simulink model "Closedloop"  (R2015b)
settings: Solver=VariableStepAuto  StartTime=0.0  StopTime=100  FixedStep=0.0001  RelTol=1e-6
values from neighbouring files (symbols this model uses):
  A = [a11 a12 a13;a21 a22 a23;a31 a32 a33]    [ControllerWT1.m]    (also in ControllerWT2.m; Robustness.m)
  B = [b11*10^6 b12*10^4;b21*10^6 b22*10^4;b31*10^6 b32*10^4]    [ControllerWT1.m]    (also in ControllerWT2.m; Robustness.m = [0 b11*10^6 b12*10^4;0 b21*10^6 b22*10^4;0 b31*10^6 b32*10^4)
  C = [0 0 0;1 0 0;a21 a22 a23;0 0 0;0 1 0]    [ControllerWT1.m]    (also in ControllerWT2.m; Robustness.m = [0 0 0;1 0 0;a21 a22 a23;1 0 0;0 0 0;0 1 0])
  Cp = xlsread(filename)    [Run_me.m]
  D = [0 1;0 0;b21*10^6 b22*10^4;1 0;0 0]    [ControllerWT1.m]    (also in ControllerWT2.m; Robustness.m = [0 0 1;0 0 0;0 b21*10^6 b22*10^4;-lambda_opt/R 0 0;0 1 0;0 0)
  lambda_opt = 7.1    [ControllerWT1.m]    (also in ControllerWT2.m; Robustness.m; Run_me.m)
  R = ureal('Rho',35,'Percentage',1)    [ControllerWT1.m]    (also in ControllerWT2.m; Robustness.m = ureal('Rho',35,'Percentage',15); Run_me.m = 35)
  Rho = ureal('Rho',1.225,'Percentage',1)    [ControllerWT1.m]    (also in ControllerWT2.m; Robustness.m = ureal('Rho',1.225,'Percentage',15); Run_me.m = 1.225)
undefined symbols (not defined in the file or in its folder): OutList, strmatch
settings Model: Creator=bjonkman  LastModifiedBy=alino
settings DataIOCC: SaveFormat=Array  SignalLoggingSaveFormat=ModelDataLogs  SaveOutput=off  SaveTime=off  SignalLoggingName=sigsOut
settings OptimizationCC: ExpressionDepthLimit=2147483647
settings DebuggingCC: SaveWithParameterizedLinksMsg=none  UnderspecifiedInitializationDetection=Classic  MergeDetectMultiDrivingBlocksExec=none  SignalResolutionControl=TryResolveAllWithWarning  MultiTaskDSMMsg=warning  MultiTaskCondExecSysMsg=none  FcnCallInpInsideContextMsg=EnableAllAsWarning  StateNameClashWarn=warning
settings HardwareCC: ProdBitPerPointer=32  ProdLargestAtomicFloat=None  ProdIntDivRoundTo=Undefined  ProdEndianess=Unspecified  ProdWordSize=32  ProdHWDeviceType=32-bit Generic  TargetUnknown=on
settings GRTTargetCC: GeneratePreprocessorConditionals=Disable all  CombineOutputUpdateFcns=off  GRTInterface=on
settings ConfigComp: CovModelRefEnable=Off

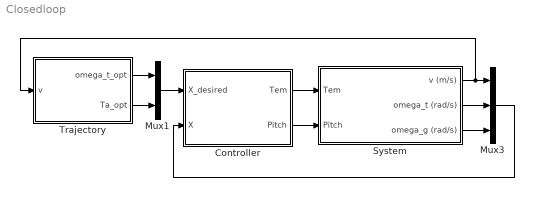
== system Closedloop ==
  Controller : Subsystem
  Mux1 : Mux  Inputs=2
  Mux3 : Mux  Inputs=3
  System : Subsystem
  Trajectory : Subsystem
  wires:
  Mux3/1 -> Controller/2(X)
  Mux1/1 -> Controller/1(X_desired)
  Trajectory/1(omega_t_opt) -> Mux1/1
  Controller/1(Tem) -> System/1(Tem)
  Controller/2(Pitch) -> System/2(Pitch)
  System/3(omega_g (rad/s)) -> Mux3/3
  System/2(omega_t (rad/s)) -> Mux3/2
  System/1(v (m/s)) -> Mux3/1, Trajectory/1(v)
  Trajectory/2(Ta_opt) -> Mux1/2

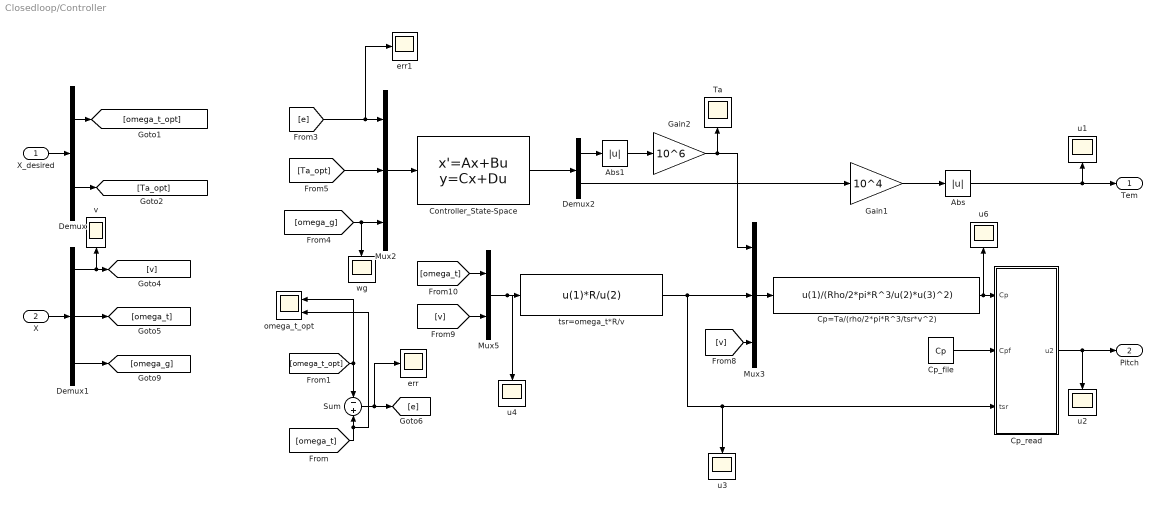
== system Closedloop/Controller ==
  X_desired : Inport
  X : Inport  Port=2
  Abs : Abs
  Abs1 : Abs
  Controller_State-Space : StateSpace  A=A  B=B  C=C  D=D  X0=0
  Cp=Ta/(rho/2*pi*R^3/tsr*v^2) : Fcn  Expr=u(1)/(Rho/2*pi*R^3/u(2)*u(3)^2)
  Cp_file : Constant  Value=Cp
  Cp_read : MATLAB Function  TreatAsAtomicUnit=on
  Demux : Demux  Outputs=2
  Demux1 : Demux  Outputs=3
  Demux2 : Demux  Outputs=2
  Gain1 : Gain  Gain=10^4
  Gain2 : Gain  Gain=10^6
  Mux2 : Mux  Inputs=3
  Mux3 : Mux  Inputs=3
  Mux5 : Mux  Inputs=2
  Sum : Sum  Inputs=-+
  Ta : Scope
  err : Scope
  err1 : Scope
  omega_t_opt : Scope  NumInputPorts=2
  tsr=omega_t*R/v : Fcn  Expr=u(1)*R/u(2)
  u{1..4,6} (5 alike) : Scope
  v : Scope
  wg : Scope
  Tem : Outport
  Pitch : Outport  Port=2
  wires:
  X_desired/1 -> Demux/1
  X/1 -> Demux1/1
  Demux/1 -> [omega_t_opt]
  Demux/2 -> [Ta_opt]
  Demux1/1 -> v/1, [v]
  Demux1/2 -> [omega_t]
  Demux1/3 -> [omega_g]
  Cp_read/1(u2) -> u2/1, Pitch/1
  Sum/1 -> err/1, [e]
  [omega_t] -> omega_t_opt/2, Sum/2
  [omega_t_opt] -> omega_t_opt/1, Sum/1
  [v] -> Mux3/3
  Mux5/1 -> u4/1, tsr=omega_t*R/v/1
  [v] -> Mux5/2
  [omega_t] -> Mux5/1
  tsr=omega_t*R/v/1 -> Cp_read/3(tsr), u3/1, Mux3/2
  [omega_g] -> wg/1, Mux2/3
  [Ta_opt] -> Mux2/2
  Controller_State-Space/1 -> Demux2/1
  Gain2/1 -> Ta/1, Mux3/1
  Mux3/1 -> Cp=Ta/(rho/2*pi*R^3/tsr*v^2)/1
  Cp=Ta/(rho/2*pi*R^3/tsr*v^2)/1 -> u6/1, Cp_read/1(Cp)
  Cp_file/1 -> Cp_read/2(Cpf)
  Abs/1 -> u1/1, Tem/1
  [e] -> err1/1, Mux2/1
  Demux2/1 -> Abs1/1
  Demux2/2 -> Gain1/1
  Mux2/1 -> Controller_State-Space/1
  Gain1/1 -> Abs/1
  Abs1/1 -> Gain2/1

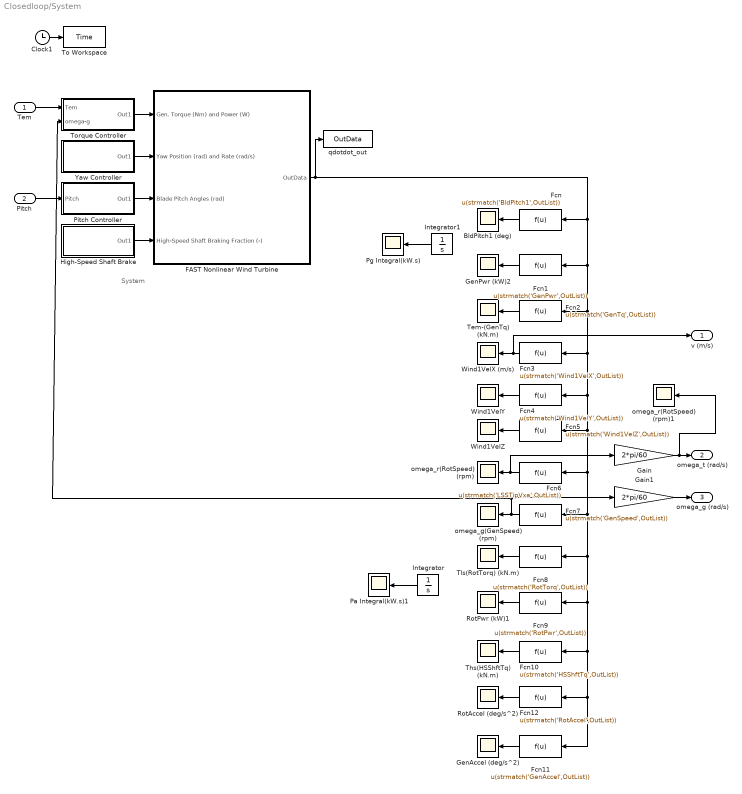
== system Closedloop/System ==
  note: System
  Tem : Inport
  Pitch : Inport  Port=2
  BldPitch1 (deg) : Scope
  Clock1 : Clock
  FAST Nonlinear Wind Turbine : Subsystem  mask(FAST Nonlinear Wind Turbine){}
      mask help: This block contains the FAST S-Function.
      mask init:
      | clear FAST_SFunc
  Fcn : Fcn  Expr=u(strmatch('BldPitch1',OutList))
  Fcn1 : Fcn  Expr=u(strmatch('GenPwr',OutList))
  Fcn10 : Fcn  Expr=u(strmatch('HSShftTq',OutList))
  Fcn11 : Fcn  Expr=u(strmatch('GenAccel',OutList))
  Fcn12 : Fcn  Expr=u(strmatch('RotAccel',OutList))
  Fcn2 : Fcn  Expr=u(strmatch('GenTq',OutList))
  Fcn3 : Fcn  Expr=u(strmatch('Wind1VelX',OutList))
  Fcn4 : Fcn  Expr=u(strmatch('Wind1VelY',OutList))
  Fcn5 : Fcn  Expr=u(strmatch('Wind1VelZ',OutList))
  Fcn6 : Fcn  Expr=u(strmatch('LSSTipVxa',OutList))
  Fcn7 : Fcn  Expr=u(strmatch('GenSpeed',OutList))
  Fcn8 : Fcn  Expr=u(strmatch('RotTorq',OutList))
  Fcn9 : Fcn  Expr=u(strmatch('RotPwr',OutList))
  Gain : Gain  Gain=2*pi/60
  Gain1 : Gain  Gain=2*pi/60
  GenAccel (deg/s^2) : Scope
  GenPwr (kW)2 : Scope
  High-Speed Shaft Brake : Subsystem
  Integrator : Integrator
  Integrator1 : Integrator
  Pa Integral(kW.s)1 : Scope
  Pg Integral(kW.s) : Scope
  Pitch Controller : Subsystem
  RotAccel (deg/s^2) : Scope
  RotPwr (kW)1 : Scope
  Tem-(GenTq) (kN.m) : Scope
  Ths(HSShftTq) (kN.m) : Scope
  Tls(RotTorq) (kN.m) : Scope
  To Workspace : ToWorkspace  VariableName=Time  SampleTime=-1
  Torque Controller : Subsystem
  Wind1VelX (m/s) : Scope
  Wind1VelY : Scope
  Wind1VelZ : Scope
  Yaw Controller : Subsystem
  omega_g(GenSpeed) (rpm) : Scope
  omega_r(RotSpeed) (rpm) : Scope
  omega_r(RotSpeed) (rpm)1 : Scope
  qdotdot_out : ToWorkspace  VariableName=OutData  SampleTime=-1
  v (m/s) : Outport
  omega_t (rad/s) : Outport  Port=2
  omega_g (rad/s) : Outport  Port=3
  wires:
  Clock1/1 -> To Workspace/1
  Torque Controller/1(Out1) -> FAST Nonlinear Wind Turbine/1(Gen. Torque (Nm) and Power (W))
  Yaw Controller/1(Out1) -> FAST Nonlinear Wind Turbine/2(Yaw Position (rad) and Rate (rad/s))
  Pitch Controller/1(Out1) -> FAST Nonlinear Wind Turbine/3(Blade Pitch Angles (rad))
  High-Speed Shaft Brake/1(Out1) -> FAST Nonlinear Wind Turbine/4(High-Speed Shaft Braking Fraction (-))
  Fcn/1 -> BldPitch1 (deg)/1
  Fcn2/1 -> Tem-(GenTq) (kN.m)/1
  Fcn3/1 -> v (m/s)/1, Wind1VelX (m/s)/1
  Fcn4/1 -> Wind1VelY/1
  Fcn5/1 -> Wind1VelZ/1
  Fcn6/1 -> Gain/1, omega_r(RotSpeed) (rpm)/1
  Fcn7/1 -> Torque Controller/2(omega-g), Gain1/1, omega_g(GenSpeed) (rpm)/1
  Fcn8/1 -> Tls(RotTorq) (kN.m)/1
  Fcn9/1 -> RotPwr (kW)1/1
  Fcn10/1 -> Ths(HSShftTq) (kN.m)/1
  Fcn12/1 -> RotAccel (deg/s^2)/1
  FAST Nonlinear Wind Turbine/1(OutData) -> Fcn11/1, Fcn12/1, Fcn10/1, Fcn9/1, Fcn8/1, Fcn7/1, Fcn6/1, Fcn5/1, Fcn4/1, Fcn3/1, Fcn2/1, Fcn1/1, Fcn/1, qdotdot_out/1
  Fcn11/1 -> GenAccel (deg/s^2)/1
  Tem/1 -> Torque Controller/1(Tem)
  Gain/1 -> omega_r(RotSpeed) (rpm)1/1, omega_t (rad/s)/1
  Gain1/1 -> omega_g (rad/s)/1
  Pitch/1 -> Pitch Controller/1(Pitch)
  Integrator/1 -> Pa Integral(kW.s)1/1
  Fcn1/1 -> GenPwr (kW)2/1
  Integrator1/1 -> Pg Integral(kW.s)/1

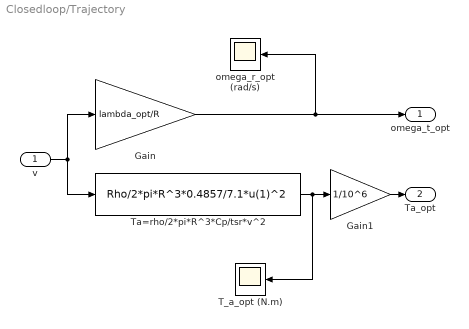
== system Closedloop/Trajectory ==
  v : Inport
  Gain : Gain  Gain=lambda_opt/R
  Gain1 : Gain  Gain=1/10^6
  T_a_opt (N.m) : Scope
  Ta=rho/2*pi*R^3*Cp/tsr*v^2 : Fcn  Expr=Rho/2*pi*R^3*0.4857/7.1*u(1)^2
  omega_r_opt (rad/s) : Scope
  omega_t_opt : Outport
  Ta_opt : Outport  Port=2
  wires:
  v/1 -> Gain/1, Ta=rho/2*pi*R^3*Cp/tsr*v^2/1
  Gain/1 -> omega_r_opt (rad/s)/1, omega_t_opt/1
  Gain1/1 -> Ta_opt/1
  Ta=rho/2*pi*R^3*Cp/tsr*v^2/1 -> T_a_opt (N.m)/1, Gain1/1

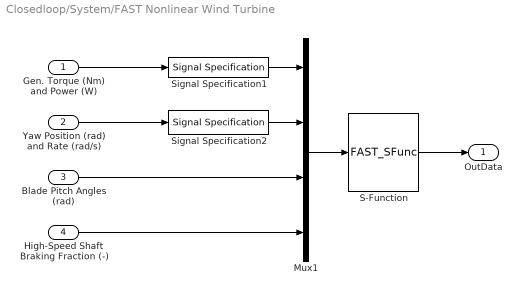
== system Closedloop/System/FAST Nonlinear Wind Turbine ==
  Gen. Torque (Nm) and Power (W) : Inport
  Yaw Position (rad) and Rate (rad/s) : Inport  Port=2
  Blade Pitch Angles (rad) : Inport  Port=3
  High-Speed Shaft Braking Fraction (-) : Inport  Port=4
  Mux1 : Mux
  S-Function : S-Function  FunctionName=FAST_SFunc  Parameters=FAST_InputFileName, TMax, 0  SFunctionDeploymentMode=off  EnableBusSupport=off
  Signal Specification1 : SignalSpecification  OutDataTypeStr=double  Dimensions=2
  Signal Specification2 : SignalSpecification  OutDataTypeStr=double  Dimensions=2
  OutData : Outport
  wires:
  Gen. Torque (Nm) and Power (W)/1 -> Signal Specification1/1
  S-Function/1 -> OutData/1
  Mux1/1 -> S-Function/1
  Blade Pitch Angles (rad)/1 -> Mux1/3
  Yaw Position (rad) and Rate (rad/s)/1 -> Signal Specification2/1
  Signal Specification1/1 -> Mux1/1
  Signal Specification2/1 -> Mux1/2
  High-Speed Shaft Braking Fraction (-)/1 -> Mux1/4

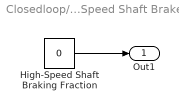
== system Closedloop/System/High-Speed Shaft Brake ==
  High-Speed Shaft Braking Fraction : Constant  Value=0
  Out1 : Outport
  wires:
  High-Speed Shaft Braking Fraction/1 -> Out1/1

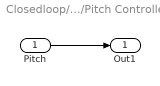
== system Closedloop/System/Pitch Controller ==
  Pitch : Inport
  Out1 : Outport
  wires:
  Pitch/1 -> Out1/1

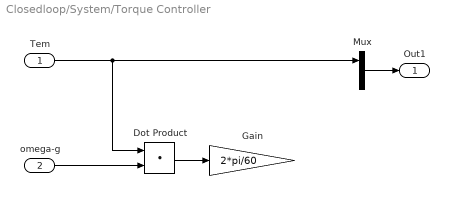
== system Closedloop/System/Torque Controller ==
  Tem : Inport
  omega-g : Inport  Port=2
  Dot Product : DotProduct  InputSameDT=on  OutDataTypeStr=Inherit: Inherit via internal rule
  Gain : Gain  Gain=2*pi/60
  Mux : Mux  Inputs=2
  Out1 : Outport
  wires:
  Mux/1 -> Out1/1
  Tem/1 -> Dot Product/1, Mux/1
  omega-g/1 -> Dot Product/2
  Dot Product/1 -> Gain/1

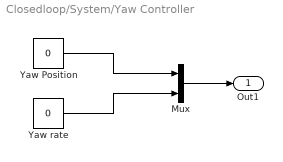
== system Closedloop/System/Yaw Controller ==
  Mux : Mux  Inputs=2
  Yaw Position : Constant  Value=0
  Yaw rate : Constant  Value=0
  Out1 : Outport
  wires:
  Mux/1 -> Out1/1
  Yaw Position/1 -> Mux/1
  Yaw rate/1 -> Mux/2

== matlab function Closedloop/Controller/Cp_read ==
  data: Cp input; u2 output; Cpf input; tsr input
function u2 = fcn(Cp,Cpf,tsr)
    tsr=floor(tsr*10+0.5);
    beta=2;
    if (Cp>0) && (Cp<0.4857) && (tsr<20) && (tsr>0)
        i=90;
        while (Cp>Cpf(i,tsr))
            i=i-1;
            if i==0 
                break; 
            end
        end
        if i~=0
            p=(Cp-Cpf(i+1,tsr))/(Cpf(i,tsr)-Cpf(i+1,tsr));
            beta=(i-p);
        end
    end
    u2=[beta,beta,beta]*pi/180;
end
